simulink library "Collector_Unglazed_ISO9806"  (R2018b)
settings: Solver=ode45  StartTime=0.0  StopTime=10.0  RelTol=1e-3  EnableMultiTasking=on
undefined symbols (not defined in the file): MassFlow, Temperature
libraries: carnot x3
settings Model: Creator=drhf  LastModifiedBy=drhf
settings DataIOCC: LimitDataPoints=on  SaveFormat=Array  SignalLoggingSaveFormat=ModelDataLogs
settings OptimizationCC: ExpressionDepthLimit=2147483647  LifeSpan=inf
settings DebuggingCC: UnderspecifiedInitializationDetection=Classic  MergeDetectMultiDrivingBlocksExec=none  SolverPrmCheckMsg=warning  FcnCallInpInsideContextMsg=warning  StateNameClashWarn=warning  SFUnexpectedBacktrackingDiag=warning  SFNoUnconditionalDefaultTransitionDiag=warning  SFExecutionAtInitializationDiag=none
settings HardwareCC: ProdBitPerPointer=32  ProdBitPerSizeT=32  ProdBitPerPtrDiffT=32  ProdLargestAtomicFloat=None  ProdIntDivRoundTo=Undefined  ProdEndianess=Unspecified  ProdWordSize=32  ProdHWDeviceType=32-bit Generic
settings ModelReferenceCC: PropagateSignalLabelsOutOfModel=off
settings SFSimCC: SimUseLocalCustomCode=off
settings RTWCC: RTWUseLocalCustomCode=off
settings CodeAppCC: StateflowObjectComments=on
settings GRTTargetCC: TargetLangStandard=C89/C90 (ANSI)  GeneratePreprocessorConditionals=Disable all  CombineOutputUpdateFcns=off  GRTInterface=on
settings ConfigComp: CovMetricSettings=dw  CovHtmlReporting=on  CovSaveCumulativeToWorkspaceVar=on  CovSaveSingleToWorkspaceVar=on  CovExternalEMLEnable=off

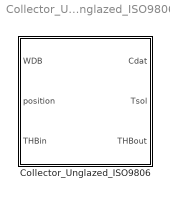
== system Collector_Unglazed_ISO9806 ==
  Collector_Unglazed_ISO9806 : Subsystem  mask(Unglazed solar thermal collector){tini=1, Ncollector=2, PathName='current', FileName='Viessmann_SLK_ISO9806_lowCp.mat', userPath=off, userParam=off, acol=2.544, len=2.1, eta0=0.702, bu=0.066, b1=32.64, b2=3.59, c_abs=2*3900, dplin=5504.4, dpqua=6222.096}
      mask prompts: tini "Initial temperature [°C]"; Ncollector "Number of collectors in parallel"; PathName "Path"; FileName "Parameter set"; userPath "Edit path and name of parameter set"; userParam "User defined parameters"; acol "Collector surface (aperture) in [m²]"; len "Length between inlet and outlet [m]"; eta0 "Optical efficiency Eta0 [-]"; bu "bu: wind dependancy of optical efficiency in W/(m²*m/s)"; b1 "b1: heat transfer for losses [W/(m²*K)]"; b2 "b2: wind dependent heat transfer for losses [W/(m²*K*m/s)]"; c_abs "Effective heat capacity of absorber [J/(m²*K)]"; dplin "Linear pressure drop in Pa/(kg/s)"; dpqua "Quadratic pressure drop in Pa/(kg/s)²"
      mask help:
      | ISO 9806 model of an unglazed solar thermal collector.
      |  Qdot = A*G*(eta0*(1-bu*vwind) - (b1 + b2*vwind)*(Tm-Tamb)/G)
      |  Qdot = mdot*cp*(Tout-Tin)
      |  Tm = (Tout+Tin)/2
      |  Tout = 2*Tm - Tin
      |  CapAbs*dTm/dt = -mdot*cp*(Tout-Tin)/A + (G*eta0*(1-bu*vwind) - (b1 + b2*vwind)*(Tm-Tamb))
      | Keep in mind that the ISO equation is not respecting the energy conservation for variable inlet conditions (e.g. temperature).
      | IT IS RECOMMENDED TO USE THIS MODEL ONLY FOR STEADY STATE CONDITIONS AT THE INLET (use Collector_Unglazed_ISO_2node model for system simulation).
      mask init:
      | [ok, param] = CarnotCallbacks_CollectorUnglazedConf('SetParameters',gcbh,PathName,FileName);
      mask Help: web(fullfile(path_carnot('help'),'Collector_Unglazed_ISO9806.html'),'-helpbrowser')
      mask TypeOptions tini: Integrator/InitialCondition
      mask TypeOptions Ncollector: ncol/Gain | ncol1/Gain | Constant/Value
      mask Callback userPath: [ok, param] = CarnotCallbacks_CollectorUnglazedISO9806('UserEdit',gcbh);
      mask Callback userParam: [ok, param] = CarnotCallbacks_CollectorUnglazedISO9806('UserEdit',gcbh);
      mask TypeOptions acol: acol/Value | acol1/Value
      mask TypeOptions len: Pressure_Drop_Collector/len
      mask TypeOptions eta0: eta0/Gain
      mask TypeOptions bu: bu/Gain
      mask TypeOptions b1: b1/Bias
      mask TypeOptions b2: b2/Gain
      mask TypeOptions c_abs: c_abs/Value
      mask TypeOptions dplin: Pressure_Drop_Collector/lin
      mask TypeOptions dpqua: Pressure_Drop_Collector/qua
      mask DialogControl Container7 Prompt: Calculation
      mask DialogControl ParameterGroupVar Prompt: Picking a parameter set
      mask DialogControl Control3 Prompt: Carnot public data
      mask DialogControl Control3 Callback: [ok, file] = CarnotCallbacks_CollectorUnglazedISO9806('GetFilename',gcbh, 'public');
      mask DialogControl Control4 Prompt: Carnot internal data
      mask DialogControl Control4 Callback: [ok, file] = CarnotCallbacks_CollectorUnglazedISO9806('GetFilename',gcbh, 'internal');
      mask DialogControl Control2 Prompt: Selected path
      mask DialogControl Control2 Callback: [ok, file] = CarnotCallbacks_CollectorUnglazedISO9806('GetFilename',gcbh, 'selected');
      mask DialogControl Container9 Prompt: Parameter values
      mask DialogControl Container8 Prompt: Geometry
      mask DialogControl Container11 Prompt: Thermal
      mask DialogControl Container12 Prompt: Hydraulic
      mask DialogControl Control6 Prompt: Save in Carnot internal data
      mask DialogControl Control6 Callback: [ok, param] = CarnotCallbacks_CollectorUnglazedISO9806('SaveFilename',gcbh, 'internal','USTC');
      mask DialogControl Control5 Prompt: Save in selected path
      mask DialogControl Control5 Callback: [ok, param] = CarnotCallbacks_CollectorUnglazedISO9806('SaveFilename',gcbh, 'selected','USTC');
      mask Display:
      | % user defined picture file
      | picfile = fullfile(path_carnot('intlibsl'), ...
      |     'Source','Solar_Thermal','Collector_Unglazed_ISO9806','parameter_set','Collector_CONF.jpg');
      | 
      | pic = false;
      | 
      | % show internal picture if defined
      | if ~BlockIsInCarnotLibrary    % if not located in library any more
      |     if exist(picfile)
      |         image(imread(picfile), [0.2, 0, 0.6, 1])
      |         set_param(gcb, 'BackgroundColor', 'White')
      |         pic = true;
      |     end
      | end
      | 
      | if ~pic % show public picture
      |     disp('ISO 9806 unglazed\n\n\n\n\n\n\n\n\n\n')
      |     plot([0,70,70,0,0]/140+0.1,         [-0,-0,5,5,-0]/140+0.1, ...
      |         [30,30,100,100,30]/140+0.1,     [100,94,94,100,100]/140+0.1, ...
      |         [32,1]/140+0.1,                 [94,5]/140+0.1, ...
      |         [40,10]/140+0.1,                [94,5]/140+0.1, ...
      |         [49,19]/140+0.1,                [94,5]/140+0.1, ...
      |         [57,27]/140+0.1,                [94,5]/140+0.1, ...
      |         [65,35]/140+0.1,                [94,5]/140+0.1, ...
      |         [73,43]/140+0.1,                [94,5]/140+0.1, ...
      |         [82,51]/140+0.1,                [94,5]/140+0.1, ...
      |         [90,60]/140+0.1,                [94,5]/140+0.1,...
      |         [98,68]/140+0.1,                [94,5]/140+0.1)
      |     set_param(gcb, 'BackgroundColor', 'Yellow')
      | end

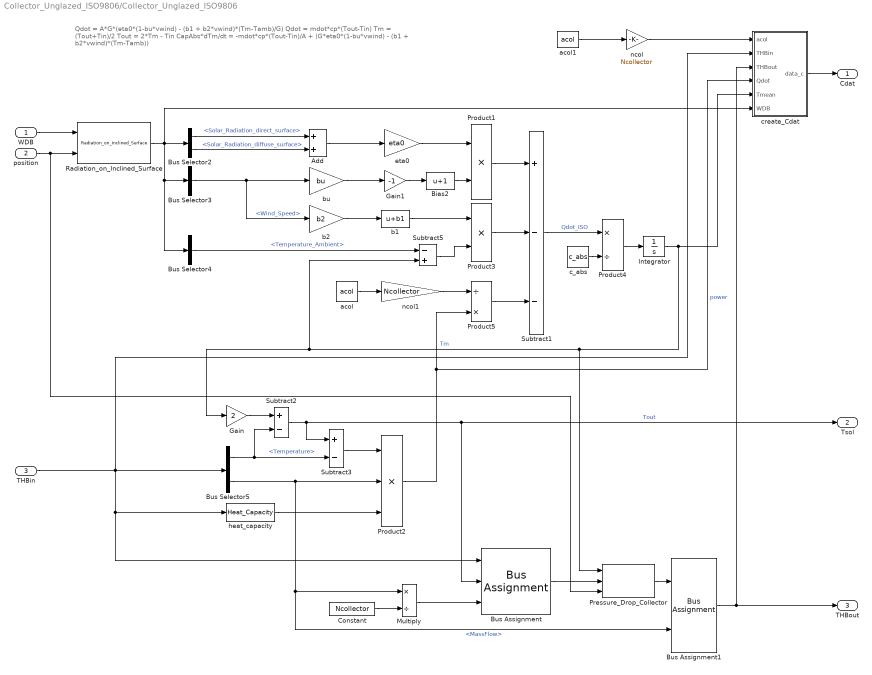
== system Collector_Unglazed_ISO9806/Collector_Unglazed_ISO9806 ==
  note: Qdot = A*G*(eta0*(1-bu*vwind) - (b1 + b2*vwind)*(Tm-Tamb)/G)
      | Qdot = mdot*cp*(Tout-Tin)
      | Tm = (Tout+Tin)/2
      | Tout = 2*Tm - Tin
      | CapAbs*dTm/dt = -mdot*cp*(Tout-Tin)/A + (G*eta0*(1-bu*vwind) - (b1 + b2*vwind)*(Tm-Tamb))
  WDB : Inport
  position : Inport  Port=2
  THBin : Inport  Port=3
  Add : Sum  Inputs=2
  Bias2 : Bias  Bias=1
  Bus Assignment : BusAssignment  AssignedSignals=Temperature,MassFlow
  Bus Assignment1 : BusAssignment  AssignedSignals=MassFlow
  Bus Selector2 : BusSelector  OutputSignals=Solar_Radiation_direct_surface,Solar_Radiation_diffuse_surface
  Bus Selector3 : BusSelector  OutputSignals=Wind_Speed
  Bus Selector4 : BusSelector  OutputSignals=Temperature_Ambient
  Bus Selector5 : BusSelector  OutputSignals=Temperature,MassFlow
  Constant : Constant  Value=Ncollector
  Gain : Gain  Gain=2
  Gain1 : Gain  Gain=-1
  Integrator : Integrator  InitialCondition=tini
  Multiply : Product  Inputs=*/
  Pressure_Drop_Collector : carnot/Basic/Pressure_Drop/Pressure_Drop_Collector  len=len  lin=dplin  qua=dpqua
      settings: SourceProductName=Carnot
  Product1 : Product  RndMeth=Zero
  Product2 : Product  Inputs=3  RndMeth=Zero
  Product3 : Product  RndMeth=Zero
  Product4 : Product  Inputs=*/  RndMeth=Zero
  Product5 : Product  Inputs=/*  RndMeth=Zero
  Radiation_on_Inclined_Surface : carnot/Weather/Radiation_on_Inclined_Surface  sky=Perez 1990  reflect=0.2
      settings: SourceProductName=Carnot
  Subtract1 : Sum  Inputs=+--
  Subtract2 : Sum  Inputs=+-
  Subtract3 : Sum  Inputs=+-
  Subtract5 : Sum  Inputs=-+
  acol : Constant  Value=acol
  acol1 : Constant  Value=acol
  b1 : Bias  Bias=b1
  b2 : Gain  Gain=b2
  bu : Gain  Gain=bu
  c_abs : Constant  Value=c_abs
  create_Cdat : Subsystem
  eta0 : Gain  Gain=eta0
  heat_capacity : carnot/Basic/Material_Properties/Heat_Capacity  VariantControl=CarlibClassic  INPUTARGUMENTS=THB  DEBUGLEVEL=DEBUGLEVEL  MAXTOTALWARNINGS=inf  MAXCONSECUTIVEWARNINGS=inf  WRITETOFILE=0  FILENAME='errors.txt'
      settings: SourceProductName=Carnot
  ncol : Gain  Gain=Ncollector
  ncol1 : Gain  Gain=Ncollector
  Cdat : Outport
  Tsol : Outport  Port=2
  THBout : Outport  Port=3  InitialOutput=0
  wires:
  Gain1/1 -> Bias2/1
  ncol1/1 -> Product5/1
  ncol/1 -> create_Cdat/1(acol)
  Bus Assignment/1 -> Pressure_Drop_Collector/2
  Pressure_Drop_Collector/1 -> Bus Assignment1/1
  bu/1 -> Gain1/1
  acol/1 -> ncol1/1
  c_abs/1 -> Product4/2
  position/1 -> Radiation_on_Inclined_Surface/2, Pressure_Drop_Collector/3
  acol1/1 -> ncol/1
  Subtract1/1 -> Product4/1  "Qdot_ISO"
  Product4/1 -> Integrator/1
  create_Cdat/1(data_c) -> Cdat/1
  WDB/1 -> Radiation_on_Inclined_Surface/1
  Product2/1 -> Product5/2, create_Cdat/4(Qdot)  "power"
  Subtract3/1 -> Product2/1
  Subtract2/1 -> Tsol/1, Bus Assignment/2, Subtract3/1  "Tout"
  Bus Selector5/2 -> Bus Assignment1/2, Multiply/1, Product2/2  "<MassFlow>"
  Product5/1 -> Subtract1/3
  Radiation_on_Inclined_Surface/1 -> Bus Selector2/1, Bus Selector4/1, Bus Selector3/1, create_Cdat/6(WDB)
  Gain/1 -> Subtract2/1
  Bias2/1 -> Product1/2
  Add/1 -> eta0/1
  b1/1 -> Product3/1
  Bus Selector3/1 -> b2/1, bu/1  "<Wind_Speed>"
  Subtract5/1 -> Product3/2
  eta0/1 -> Product1/1
  Product3/1 -> Subtract1/2
  b2/1 -> b1/1
  THBin/1 -> Bus Selector5/1, heat_capacity/1, Bus Assignment/1, create_Cdat/2(THBin)
  heat_capacity/1 -> Product2/3
  Bus Selector2/2 -> Add/2  "<Solar_Radiation_diffuse_surface>"
  Bus Selector5/1 -> Subtract3/2, Subtract2/2  "<Temperature>"
  Bus Selector2/1 -> Add/1  "<Solar_Radiation_direct_surface>"
  Bus Selector4/1 -> Subtract5/1  "<Temperature_Ambient>"
  Product1/1 -> Subtract1/1
  Integrator/1 -> Gain/1, Subtract5/2, Pressure_Drop_Collector/1, create_Cdat/5(Tmean)  "Tm"
  Constant/1 -> Multiply/2
  Multiply/1 -> Bus Assignment/3
  Bus Assignment1/1 -> THBout/1, create_Cdat/3(THBout)

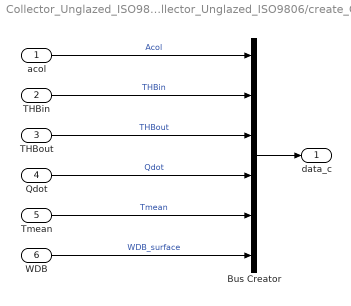
== system Collector_Unglazed_ISO9806/Collector_Unglazed_ISO9806/create_Cdat ==
  acol : Inport
  THBin : Inport  Port=2
  THBout : Inport  Port=3
  Qdot : Inport  Port=4
  Tmean : Inport  Port=5
  WDB : Inport  Port=6
  Bus Creator : BusCreator  Inputs=6
  data_c : Outport
  wires:
  acol/1 -> Bus Creator/1  "Acol"
  THBin/1 -> Bus Creator/2  "THBin"
  THBout/1 -> Bus Creator/3  "THBout"
  WDB/1 -> Bus Creator/6  "WDB_surface"
  Bus Creator/1 -> data_c/1
  Qdot/1 -> Bus Creator/4  "Qdot"
  Tmean/1 -> Bus Creator/5  "Tmean"
